simulink model "massanddamper"  (R2020b)
settings: Solver=VariableStepAuto  StartTime=0.0  StopTime=10.0  RelTol=1e-3
undefined symbols (not defined in the file): B, K, m
settings Model: Creator=Raana  LastModifiedBy=Raana
settings DataIOCC: ReturnWorkspaceOutputs=off

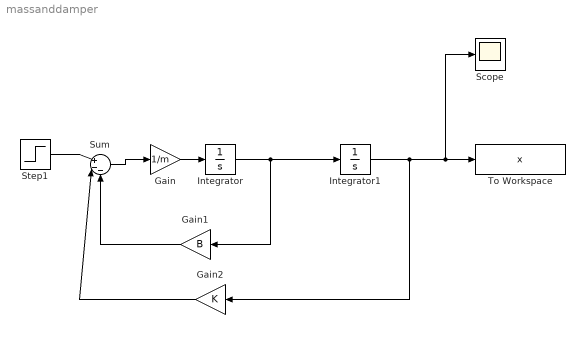
== system massanddamper ==
  Gain : Gain  Gain=1/m
  Gain1 : Gain  Gain=B
  Gain2 : Gain  Gain=K
  Integrator : Integrator
  Integrator1 : Integrator
  Scope : Scope
  Step1 : Step  After=5  SampleTime=0
  Sum : Sum  Inputs=|+--
  To Workspace : ToWorkspace  VariableName=x  SampleTime=-1
  wires:
  Integrator/1 -> Gain1/1, Integrator1/1
  Gain/1 -> Integrator/1
  Step1/1 -> Sum/1
  Sum/1 -> Gain/1
  Integrator1/1 -> Gain2/1, Scope/1, To Workspace/1
  Gain2/1 -> Sum/2
  Gain1/1 -> Sum/3
